simulink model "refresh_active_vessel"  (R2020a)
settings: Solver=FixedStepDiscrete  StartTime=0.0  StopTime=10.0  RelTol=1e-3
settings Model: Creator=thomas  LastModifiedBy=thomas

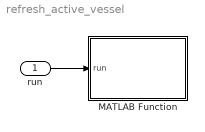
== system refresh_active_vessel ==
  run : Inport  OutDataTypeStr=boolean
  MATLAB Function : MATLAB Function  TreatAsAtomicUnit=on
  wires:
  run/1 -> MATLAB Function/1(run)

== matlab function refresh_active_vessel/MATLAB Function ==
  data: run input
function read_state(run)
    coder.extrinsic('evalin');
    if run
        evalin('base', 'vessel = spaceCenter.getActiveVessel();');
        evalin('base', 'vessel_control = vessel.getControl();');
        evalin('base', 'vessel_surface_rf = vessel.getSurfaceReferenceFrame();');
        evalin('base', 'vessel_regular_rf = vessel.getReferenceFrame();');
        evalin('base', 'vessel_orbital_rf = vessel.getOrbitalReferenceFrame();');
        evalin('base', 'vessel_flight = vessel.flight(vessel_surface_rf);');
        evalin('base', 'vessel_flight_rf = vessel.flight(vessel_regular_rf);');
        evalin('base', 'vessel_orbit = vessel.getOrbit();');
        evalin('base', 'autoPilot = vessel.getAutoPilot();');
    end
end
